simulink model "Scenario_17_v2"  (R2020b)
settings: Solver=ode1  StartTime=0.0  StopTime=10  FixedStep=Ts  MaxStep=Ts  MinStep=Ts/50  RelTol=1e-3
values from neighbouring files (symbols this model uses):
  c0 = c0_zeb    (= 6.57988e-09)    [Scenario_17_parameters_v2.m]    (also in Scenario_1_parameters_v2.m; Scenario_2_parameters_v2.m; Scenario_3_parameters_v2.m)
  c1 = c1_zeb    (= 9.15905e-09)    [Scenario_17_parameters_v2.m]    (also in Scenario_1_parameters_v2.m; Scenario_2_parameters_v2.m; Scenario_3_parameters_v2.m)
  fg = 50    [Scenario_17_parameters_v2.m]    (also in Scenario_1_parameters_v2.m; Scenario_2_parameters_v2.m; Scenario_3_parameters_v2.m)
  G11gen = 0.50    (= 0.5)    [Scenario_17_parameters_v2.m]
  G1gen = 0.4692    [Scenario_17_parameters_v2.m]    (also in Scenario_1_parameters_v2.m = 0.1; Scenario_2_parameters_v2.m = 0.298581; Scenario_3_parameters_v2.m = 0.65)
  G5gen = 0.75    [Scenario_17_parameters_v2.m]    (also in Scenario_1_parameters_v2.m = 0.8; Scenario_2_parameters_v2.m = 0.8; Scenario_3_parameters_v2.m = 0.705)
  G6gen = 0.90    (= 0.9)    [Scenario_17_parameters_v2.m]    (also in Scenario_1_parameters_v2.m; Scenario_2_parameters_v2.m = 0.81797; Scenario_3_parameters_v2.m = 0.45)
  G7gen = 0.20    (= 0.2)    [Scenario_17_parameters_v2.m]    (also in Scenario_1_parameters_v2.m = 0.5227; Scenario_2_parameters_v2.m = 0.5098; Scenario_3_parameters_v2.m = 0.4)
  G8gen = 0.58    [Scenario_17_parameters_v2.m]    (also in Scenario_3_parameters_v2.m = 0.65)
  G9gen = 0.8833    [Scenario_17_parameters_v2.m]    (also in Scenario_3_parameters_v2.m = 0.9)
  Iovc = 1.2    [Scenario_17_parameters_v2.m]    (also in Scenario_1_parameters_v2.m; Scenario_2_parameters_v2.m; Scenario_3_parameters_v2.m)
  l0 = l0_zeb    (= 0.00368)    [Scenario_17_parameters_v2.m]    (also in Scenario_1_parameters_v2.m; Scenario_2_parameters_v2.m; Scenario_3_parameters_v2.m)
  l1 = l1_zeb    (= 0.00128)    [Scenario_17_parameters_v2.m]    (also in Scenario_1_parameters_v2.m; Scenario_2_parameters_v2.m; Scenario_3_parameters_v2.m)
  L11dem = 0.02    [Scenario_17_parameters_v2.m]
  L12dem = 0.01    [Scenario_17_parameters_v2.m]    (also in Scenario_3_parameters_v2.m = 0.02)
  L1dem = 0.25    [Scenario_17_parameters_v2.m]    (also in Scenario_3_parameters_v2.m = 0.1)
  L3dem = 0.30    (= 0.3)    [Scenario_17_parameters_v2.m]    (also in Scenario_1_parameters_v2.m = 0.1; Scenario_2_parameters_v2.m = 0.1; Scenario_3_parameters_v2.m = 0.2)
  L5dem = 0.25    [Scenario_17_parameters_v2.m]    (also in Scenario_1_parameters_v2.m = 0.35; Scenario_2_parameters_v2.m = 0.35; Scenario_3_parameters_v2.m = 0.1)
  L9dem = 0.15    [Scenario_17_parameters_v2.m]    (also in Scenario_3_parameters_v2.m = 0.1)
  Pr = Sr*PF    (= 1600500000)    [Scenario_17_parameters_v2.m]    (also in Scenario_1_parameters_v2.m = 1472500000; Scenario_2_parameters_v2.m = 1805000000; Scenario_3_parameters_v2.m = 12740000000)
  Qr = sqrt(Sr^2 - Pr^2)    [Scenario_17_parameters_v2.m]    (also in Scenario_1_parameters_v2.m; Scenario_2_parameters_v2.m; Scenario_3_parameters_v2.m)
  r0 = r0_zeb    (= 0.39362)    [Scenario_17_parameters_v2.m]    (also in Scenario_1_parameters_v2.m; Scenario_2_parameters_v2.m; Scenario_3_parameters_v2.m)
  r1 = r1_zeb    (= 0.06862)    [Scenario_17_parameters_v2.m]    (also in Scenario_1_parameters_v2.m; Scenario_2_parameters_v2.m; Scenario_3_parameters_v2.m)
  Rtpu = Xtpu/40    (= 0.0025)    [Scenario_17_parameters_v2.m]    (also in Scenario_1_parameters_v2.m = 0.00375; Scenario_2_parameters_v2.m = 0.00375; Scenario_3_parameters_v2.m)
  S11non = 50e6    (= 50000000)    [Scenario_17_parameters_v2.m]
  S1non = 700e6    (= 700000000)    [Scenario_17_parameters_v2.m]    (also in Scenario_1_parameters_v2.m = 400000000; Scenario_2_parameters_v2.m = 400000000; Scenario_3_parameters_v2.m = 1000000000)
  S5non = 400e6    (= 400000000)    [Scenario_17_parameters_v2.m]    (also in Scenario_1_parameters_v2.m = 500000000; Scenario_2_parameters_v2.m = 500000000; Scenario_3_parameters_v2.m = 2000000000)
  S6non = 150e6    (= 150000000)    [Scenario_17_parameters_v2.m]    (also in Scenario_1_parameters_v2.m = 400000000; Scenario_2_parameters_v2.m = 400000000; Scenario_3_parameters_v2.m = 3000000000)
  S7non = 1500e6    (= 1500000000)    [Scenario_17_parameters_v2.m]    (also in Scenario_1_parameters_v2.m = 200000000; Scenario_2_parameters_v2.m = 200000000; Scenario_3_parameters_v2.m = 4000000000)
  S8non = 600e6    (= 600000000)    [Scenario_17_parameters_v2.m]    (also in Scenario_3_parameters_v2.m = 2000000000)
  S9non = 200e6    (= 200000000)    [Scenario_17_parameters_v2.m]    (also in Scenario_3_parameters_v2.m = 1500000000)
  tonvsc = 0    [Scenario_17_parameters_v2.m]    (also in Scenario_1_parameters_v2.m; Scenario_2_parameters_v2.m; Scenario_3_parameters_v2.m = 0.0001)
  Ts = 50e-6    (= 5e-05)    [Scenario_17_parameters_v2.m]    (also in Scenario_1_parameters_v2.m = 0.0002; Scenario_2_parameters_v2.m = 2e-05; Scenario_3_parameters_v2.m = 0.0001)
  Vhv = 220e3    (= 220000)    [Scenario_17_parameters_v2.m]    (also in Scenario_1_parameters_v2.m; Scenario_2_parameters_v2.m; Scenario_3_parameters_v2.m)
  Vmv = 22e3    (= 22000)    [Scenario_17_parameters_v2.m]    (also in Scenario_1_parameters_v2.m; Scenario_2_parameters_v2.m; Scenario_3_parameters_v2.m)
  w_pll = 2*pi*80    (= 502.654824574)    [Scenario_17_parameters_v2.m]    (also in Scenario_1_parameters_v2.m; Scenario_2_parameters_v2.m; Scenario_3_parameters_v2.m)
  wc1 = wsw1/10    (= 848.230016469)    [Scenario_17_parameters_v2.m]    (also in Scenario_1_parameters_v2.m; Scenario_2_parameters_v2.m; Scenario_3_parameters_v2.m)
  wdc1 = wc1/10    (= 84.8230016469)    [Scenario_17_parameters_v2.m]    (also in Scenario_1_parameters_v2.m; Scenario_2_parameters_v2.m; Scenario_3_parameters_v2.m)
  wpq1 = wc1/10    (= 84.8230016469)    [Scenario_17_parameters_v2.m]    (also in Scenario_1_parameters_v2.m; Scenario_2_parameters_v2.m; Scenario_3_parameters_v2.m)
  wsw1 = ksw1*2*pi*fg    (= 8482.30016469)    [Scenario_17_parameters_v2.m]    (also in Scenario_1_parameters_v2.m; Scenario_2_parameters_v2.m; Scenario_3_parameters_v2.m)
  Xtpu = 0.10    (= 0.1)    [Scenario_17_parameters_v2.m]    (also in Scenario_1_parameters_v2.m = 0.15; Scenario_2_parameters_v2.m = 0.15; Scenario_3_parameters_v2.m)
undefined symbols (not defined in the file or in its folder): D11, Delta, Newton, Raphson
libraries: powerlib x349, simulink_extras x215, powerlib_meascontrol x165, pid_lib x81, simulink x48, eeTransforms x42, spsFirstOrderFilterLib x28, eePwmGeneratorTwoLevel x7
(part 1 of 31)
settings Model: Creator=Usuario  LastModifiedBy=Usuario
settings SolverCC: InitialStep=Ts/50  MaxConsecutiveMinStep=100  ShapePreserveControl=EnableAll  ZeroCrossAlgorithm=Adaptive
settings DebuggingCC: UnconnectedInputMsg=none  UnconnectedOutputMsg=none  UnconnectedLineMsg=none

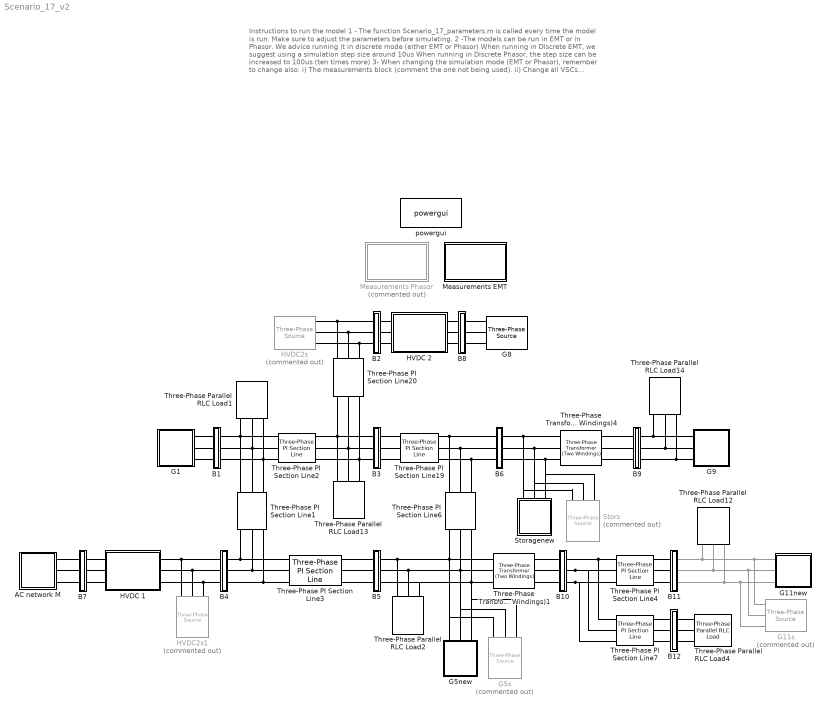
== system Scenario_17_v2 ==
  note: Instructions to run the model
      |
      | 1 - The function Scenario_17_parameters.m is called every time the model is run. Make sure to adjust the parameters before simulating.
      | 2 -The models can be run in EMT or in Phasor. We advice running it in discrete mode (either EMT or Phasor)
      | 	When running in Discrete EMT, we suggest using a simulation step size around 10us
      | 	When running in Discrete Phasor, the step size can be increased to 100us (ten times more)
      | 3- When changing the simulation mode (EMT or Phasor), remember to change also:
      | 	i) The measurements block (comment the one not being used).
      | 	ii) Change all VSCs models of blocks (G5,G11,Storage, HVDC 1 and HVDC 2).
      | 	    To change the model, go to the block VSC and choose one model of droplist under the parameter 'VSC model'
      | 	    We recommend the model AVG model for EMT and the I-ref model for Phasor.
      | 4- The synchronous generators were initialized using power flow to have a near-flat initialization.
      |      As the VSCs are not standard blocks in Simulink, they are not considered in the power flow.
      |     To consider them, connect the voltage source in their place and run the power flow. Then, substitute by the VSCs.
  AC network M : Subsystem
      mask Display: disp('SG')
  B1 : Subsystem
  B10 : Subsystem
  B11 : Subsystem
  B12 : Subsystem
  B2 : Subsystem
  B3 : Subsystem
  B4 : Subsystem
  B5 : Subsystem
  B6 : Subsystem
  B7 : Subsystem
  B8 : Subsystem
  B9 : Subsystem
  G1 : Subsystem
      mask Display:
      | disp('SG')
      | %x = [0:0.001:1];
      | %y = 0.2*sin(10*x) + 0.5;
      | %plot(x,y)
  G11new : Subsystem
  G11s : powerlib/Electrical Sources/Three-Phase Source  Commented=on  InternalConnection=Yg  VoltagePhases=off  Voltage=(22000)*1.15821  PhaseAngle=-42.2179  Voltage_phases=[25e3 25e3 25e3]/sqrt(3)  PhaseAngles_phases=[0 -120 +120]  Frequency=fg  NonIdealSource=on  SpecifyImpedance=off  Resistance=Rtpu*(Vmv^2/S11non)  Inductance=Xtpu*(Vmv^2/S11non) * 1/(2*pi*fg)  ShortCircuitLevel=Svsc1  BaseVoltage=Vmv  XRratio=Xtpu/Rtpu  BusType=PQ  Pref=S11non*G11gen  Qref=20e6  Prefabc=[10e3, 10e3, 10e3]  Qrefabc=[0, 0, 0]  Qmin=-inf  Qmax=inf
  G5new : Subsystem
  G5s : powerlib/Electrical Sources/Three-Phase Source  Commented=on  InternalConnection=Yg  VoltagePhases=off  Voltage=(220000)*1.07588  PhaseAngle=-28.957  Voltage_phases=[25e3 25e3 25e3]/sqrt(3)  PhaseAngles_phases=[0 -120 +120]  Frequency=fg  NonIdealSource=on  SpecifyImpedance=off  Resistance=Rtpu*(Vhv^2/S5non)  Inductance=Xtpu*(Vhv^2/S5non) * 1/(2*pi*fg)  ShortCircuitLevel=Svsc1  BaseVoltage=Vhv  XRratio=Xtpu/Rtpu  BusType=PQ  Pref=S5non*G5gen  Qref=150e6  Prefabc=[10e3, 10e3, 10e3]  Qrefabc=[0, 0, 0]  Qmin=-inf  Qmax=inf
  G8 : powerlib/Electrical Sources/Three-Phase Source  InternalConnection=Yg  VoltagePhases=off  Voltage=Vhv  PhaseAngle=0  Voltage_phases=[25e3 25e3 25e3]/sqrt(3)  PhaseAngles_phases=[0 -120 +120]  Frequency=fg  NonIdealSource=on  SpecifyImpedance=off  Resistance=Rtpu*(Vhv^2/S8non)  Inductance=Xtpu*(Vhv^2/S8non) * 1/(2*pi*fg)  ShortCircuitLevel=100e6  BaseVoltage=Vhv  XRratio=7  BusType=PV  Pref=S8non*G8gen  Qref=0  Prefabc=[10e3, 10e3, 10e3]  Qrefabc=[0, 0, 0]  Qmin=-inf  Qmax=inf
  G9 : Subsystem
      mask Display: disp('SG')
  HVDC 1 : Subsystem
  HVDC 2 : Subsystem
  HVDC2s : powerlib/Electrical Sources/Three-Phase Source  Commented=on  InternalConnection=Yg  VoltagePhases=off  Voltage=(220000)*0.984881  PhaseAngle=-24.9359  Voltage_phases=[25e3 25e3 25e3]/sqrt(3)  PhaseAngles_phases=[0 -120 +120]  Frequency=fg  NonIdealSource=on  SpecifyImpedance=off  Resistance=Rtpu*(Vhv^2/S8non)  Inductance=Xtpu*(Vhv^2/S8non) * 1/(2*pi*fg)  ShortCircuitLevel=Svsc1  BaseVoltage=Vhv  XRratio=Xtpu/Rtpu  BusType=PQ  Pref=S8non*G8gen  Qref=0  Prefabc=[10e3, 10e3, 10e3]  Qrefabc=[0, 0, 0]  Qmin=-inf  Qmax=inf
  HVDC2s1 : powerlib/Electrical Sources/Three-Phase Source  Commented=on  InternalConnection=Yg  VoltagePhases=off  Voltage=(220000)*1.05033  PhaseAngle=-28.8095  Voltage_phases=[25e3 25e3 25e3]/sqrt(3)  PhaseAngles_phases=[0 -120 +120]  Frequency=fg  NonIdealSource=on  SpecifyImpedance=off  Resistance=Rtpu*(Vhv^2/S7non)  Inductance=Xtpu*(Vhv^2/S7non) * 1/(2*pi*fg)  ShortCircuitLevel=Svsc1  BaseVoltage=Vhv  XRratio=Xtpu/Rtpu  BusType=PQ  Pref=S7non*G7gen  Qref=100e6  Prefabc=[10e3, 10e3, 10e3]  Qrefabc=[0, 0, 0]  Qmin=-inf  Qmax=inf
  Measurements EMT : Subsystem
  Measurements Phasor : Subsystem  Commented=on
  Storagenew : Subsystem
  Stors : powerlib/Electrical Sources/Three-Phase Source  Commented=on  InternalConnection=Yg  VoltagePhases=off  Voltage=(220000)*1.06618  PhaseAngle=-27.8909  Voltage_phases=[25e3 25e3 25e3]/sqrt(3)  PhaseAngles_phases=[0 -120 +120]  Frequency=fg  NonIdealSource=on  SpecifyImpedance=off  Resistance=Rtpu*(Vhv^2/S6non)  Inductance=Xtpu*(Vhv^2/S6non) * 1/(2*pi*fg)  ShortCircuitLevel=Svsc1  BaseVoltage=Vhv  XRratio=Xtpu/Rtpu  BusType=PQ  Pref=S6non*G6gen  Qref=80e6  Prefabc=[10e3, 10e3, 10e3]  Qrefabc=[0, 0, 0]  Qmin=-inf  Qmax=inf
  Three-Phase PI Section Line1 : powerlib/Elements/Three-Phase PI Section Line  LConnTagsString=a|b|c  RConnTagsString=A|B|C  Length=50  Frequency=fg  Resistances=[r1 r0]  Inductances="[l1  l0]"  Capacitances=[c1 c0]
  Three-Phase PI Section Line19 : powerlib/Elements/Three-Phase PI Section Line  LConnTagsString=a|b|c  RConnTagsString=A|B|C  Length=40  Frequency=fg  Resistances=[r1 r0]  Inductances="[l1  l0]"  Capacitances=[c1 c0]
  Three-Phase PI Section Line2 : powerlib/Elements/Three-Phase PI Section Line  LConnTagsString=a|b|c  RConnTagsString=A|B|C  Length=60  Frequency=fg  Resistances=[r1 r0]  Inductances="[l1  l0]"  Capacitances=[c1 c0]
  Three-Phase PI Section Line20 : powerlib/Elements/Three-Phase PI Section Line  LConnTagsString=a|b|c  RConnTagsString=A|B|C  Length=30  Frequency=fg  Resistances=[r1 r0]  Inductances="[l1  l0]"  Capacitances=[c1 c0]
  Three-Phase PI Section Line3 : powerlib/Elements/Three-Phase PI Section Line  LConnTagsString=a|b|c  RConnTagsString=A|B|C  Length=40  Frequency=fg  Resistances=[r1 r0]  Inductances="[l1  l0]"  Capacitances=[c1 c0]
  Three-Phase PI Section Line4 : powerlib/Elements/Three-Phase PI Section Line  LConnTagsString=a|b|c  RConnTagsString=A|B|C  Length=15  Frequency=fg  Resistances=[r1 r0]  Inductances="[l1  l0]"  Capacitances=[c1 c0]
  Three-Phase PI Section Line6 : powerlib/Elements/Three-Phase PI Section Line  LConnTagsString=a|b|c  RConnTagsString=A|B|C  Length=80  Frequency=fg  Resistances=[r1 r0]  Inductances="[l1  l0]"  Capacitances=[c1 c0]
  Three-Phase PI Section Line7 : powerlib/Elements/Three-Phase PI Section Line  LConnTagsString=a|b|c  RConnTagsString=A|B|C  Length=10  Frequency=fg  Resistances=[r1 r0]  Inductances="[l1  l0]"  Capacitances=[c1 c0]
  Three-Phase Parallel RLC Load1 : powerlib/Elements/Three-Phase Parallel RLC Load  LConnTagsString=A|B|C  Configuration=Y (grounded)  NominalVoltage=Vhv  Vabc=[1e3 1e3 1e3]  Vabcp=[1e3 1e3 1e3]  NominalFrequency=fg  UnbalancedPower=off  ActivePower=Pr*L1dem  InductivePower=Qr*L1dem  CapacitivePower=0  Pabc=[10e3 9e3 11e3]  QLabc=[100 90 110]  QCabc=[100 90 110]  Pabcp=[10e3 9e3 11e3]  QLabcp=[100 90 110]  QCabcp=[100 90 110]  Measurements=None  LoadType=constant Z
  Three-Phase Parallel RLC Load12 : powerlib/Elements/Three-Phase Parallel RLC Load  LConnTagsString=A|B|C  Configuration=Y (grounded)  NominalVoltage=Vmv  Vabc=[1e3 1e3 1e3]  Vabcp=[1e3 1e3 1e3]  NominalFrequency=fg  UnbalancedPower=off  ActivePower=Pr*L11dem  InductivePower=Qr*L11dem  CapacitivePower=0  Pabc=[10e3 9e3 11e3]  QLabc=[100 90 110]  QCabc=[100 90 110]  Pabcp=[10e3 9e3 11e3]  QLabcp=[100 90 110]  QCabcp=[100 90 110]  Measurements=None  LoadType=constant Z
  Three-Phase Parallel RLC Load13 : powerlib/Elements/Three-Phase Parallel RLC Load  LConnTagsString=A|B|C  Configuration=Y (grounded)  NominalVoltage=Vhv  Vabc=[1e3 1e3 1e3]  Vabcp=[1e3 1e3 1e3]  NominalFrequency=fg  UnbalancedPower=off  ActivePower=Pr*L3dem  InductivePower=Qr*L3dem  CapacitivePower=0  Pabc=[10e3 9e3 11e3]  QLabc=[100 90 110]  QCabc=[100 90 110]  Pabcp=[10e3 9e3 11e3]  QLabcp=[100 90 110]  QCabcp=[100 90 110]  Measurements=None  LoadType=constant Z
  Three-Phase Parallel RLC Load14 : powerlib/Elements/Three-Phase Parallel RLC Load  LConnTagsString=A|B|C  Configuration=Y (grounded)  NominalVoltage=Vmv  Vabc=[1e3 1e3 1e3]  Vabcp=[1e3 1e3 1e3]  NominalFrequency=fg  UnbalancedPower=off  ActivePower=Pr*L9dem  InductivePower=Qr*L9dem  CapacitivePower=0  Pabc=[10e3 9e3 11e3]  QLabc=[100 90 110]  QCabc=[100 90 110]  Pabcp=[10e3 9e3 11e3]  QLabcp=[100 90 110]  QCabcp=[100 90 110]  Measurements=None  LoadType=constant Z
  Three-Phase Parallel RLC Load2 : powerlib/Elements/Three-Phase Parallel RLC Load  LConnTagsString=A|B|C  Configuration=Y (grounded)  NominalVoltage=Vhv  Vabc=[1e3 1e3 1e3]  Vabcp=[1e3 1e3 1e3]  NominalFrequency=fg  UnbalancedPower=off  ActivePower=Pr*L5dem  InductivePower=Qr*L5dem  CapacitivePower=0  Pabc=[10e3 9e3 11e3]  QLabc=[100 90 110]  QCabc=[100 90 110]  Pabcp=[10e3 9e3 11e3]  QLabcp=[100 90 110]  QCabcp=[100 90 110]  Measurements=None  LoadType=constant Z
  Three-Phase Parallel RLC Load4 : powerlib/Elements/Three-Phase Parallel RLC Load  LConnTagsString=A|B|C  Configuration=Y (grounded)  NominalVoltage=Vmv  Vabc=[1e3 1e3 1e3]  Vabcp=[1e3 1e3 1e3]  NominalFrequency=fg  UnbalancedPower=off  ActivePower=Pr*L12dem  InductivePower=Qr*L12dem  CapacitivePower=0  Pabc=[10e3 9e3 11e3]  QLabc=[100 90 110]  QCabc=[100 90 110]  Pabcp=[10e3 9e3 11e3]  QLabcp=[100 90 110]  QCabcp=[100 90 110]  Measurements=None  LoadType=constant Z
  Three-Phase Transformer (Two Windings)1 : powerlib/Elements/Three-Phase Transformer (Two Windings)  Winding1Connection=Yg  Winding2Connection=Yg  CoreType=Three single-phase transformers  SetSaturation=off  Hysteresis=off  DataFile='hysteresis'  SetInitialFlux=off  Measurements=None  UNITS=pu  NominalPower=[2*S11non , fg ]  Winding1=[1.02*Vmv 0.001 0.04]  Winding2=[1.0*Vhv 0.001 0.04]  Rm=5000  Lm=5000  L0=0.5  Saturation=[ 0,0 ; 0.0024,1.2 ; 1.0,1.52 ]  InitialFluxes=[ 0.8 , -0.8 , 0.7 ]  BreakLoop=off  DiscreteSolver=Trapezoidal iterative  DataType=off  TransfoNumber=1
  Three-Phase Transformer (Two Windings)4 : powerlib/Elements/Three-Phase Transformer (Two Windings)  Winding1Connection=Yg  Winding2Connection=Yg  CoreType=Three single-phase transformers  SetSaturation=off  Hysteresis=off  DataFile='hysteresis'  SetInitialFlux=off  Measurements=None  UNITS=pu  NominalPower=[2*S9non , fg ]  Winding1=[1.0*Vmv 0.00125 0.05]  Winding2=[1.0*Vhv 0.00125 0.05]  Rm=5000  Lm=5000  L0=0.5  Saturation=[ 0,0 ; 0.0024,1.2 ; 1.0,1.52 ]  InitialFluxes=[ 0.8 , -0.8 , 0.7 ]  BreakLoop=off  DiscreteSolver=Trapezoidal iterative  DataType=off  TransfoNumber=1
  powergui : powerlib/powergui  Priority=1  SimulationMode=Discrete  SampleTime=Ts  frequency=fg  Iterations=50  frequencyindice=50  Pbase=100e6  ErrMax=0.0001  UnitsV=kV  UnitsW=MW  buscounter=0  FunctionMessages=off  echomessages=off  EnableUseOfTLC=off  CurrentSourceSwitches=off  DisableSnubberDevices=off  DisableRonSwitches=off  DisableVfSwitches=off  DisplayEquations=off  AutomaticDiscreteSolvers=off  SolverType=Tustin/Backward Euler (TBE)  Interpol=off  ExternalGateDelay=off  methode=off  Ts=100  x0status=blocks  SPID=on  SwTol=0  HookPort=off  NonlinearTolerance=1e-4  nMaxIteration=100  ContinueOnMaxIteration=off  RestoreLinks=warning  ResistiveCurrentMeasurement=off  Frange=[0:2:500]  Ylog=off  Xlog=on  ShowGrid=off  save=off  variable=ZData  structure=0  ZoomFFT=off  StartTime=0.0  cycles=1  DisplayStyle=1  fundamental=60  FreqAxis=off  MaxFrequency=1000  frequencyindicesteady=1  RmsSteady=2  display=off
  connections:
  B4/LConn1 -- HVDC 1/LConn1 -- HVDC2s1/RConn1
  B4/LConn2 -- HVDC2s1/RConn2 -- HVDC 1/LConn2
  B4/LConn3 -- HVDC2s1/RConn3 -- HVDC 1/LConn3
  G1/RConn1 -- B1/LConn1
  G1/RConn2 -- B1/LConn2
  G1/RConn3 -- B1/LConn3
  Three-Phase PI Section Line2/LConn1 -- Three-Phase Parallel RLC Load1/LConn1 -- Three-Phase PI Section Line1/RConn1 -- B1/RConn1
  Three-Phase PI Section Line2/LConn2 -- Three-Phase Parallel RLC Load1/LConn2 -- B1/RConn2 -- Three-Phase PI Section Line1/RConn2
  Three-Phase PI Section Line2/LConn3 -- B1/RConn3 -- Three-Phase Parallel RLC Load1/LConn3 -- Three-Phase PI Section Line1/RConn3
  Three-Phase PI Section Line3/LConn1 -- B4/RConn1 -- Three-Phase PI Section Line1/LConn1
  Three-Phase PI Section Line3/LConn2 -- B4/RConn2 -- Three-Phase PI Section Line1/LConn2
  Three-Phase PI Section Line3/LConn3 -- Three-Phase PI Section Line1/LConn3 -- B4/RConn3
  B5/LConn1 -- Three-Phase PI Section Line3/RConn1
  B5/LConn2 -- Three-Phase PI Section Line3/RConn2
  B5/LConn3 -- Three-Phase PI Section Line3/RConn3
  G5new/RConn1 -- G5s/RConn1 -- Three-Phase Transformer (Two Windings)1/RConn1 -- Three-Phase Parallel RLC Load2/LConn1 -- B5/RConn1 -- Three-Phase PI Section Line6/LConn1
  G5new/RConn2 -- G5s/RConn2 -- Three-Phase Parallel RLC Load2/LConn2 -- B5/RConn2 -- Three-Phase Transformer (Two Windings)1/RConn2 -- Three-Phase PI Section Line6/LConn2
  G5new/RConn3 -- G5s/RConn3 -- Three-Phase PI Section Line6/LConn3 -- Three-Phase Transformer (Two Windings)1/RConn3 -- Three-Phase Parallel RLC Load2/LConn3 -- B5/RConn3
  Three-Phase Transformer (Two Windings)1/LConn1 -- B10/LConn1
  Three-Phase Transformer (Two Windings)1/LConn2 -- B10/LConn2
  Three-Phase Transformer (Two Windings)1/LConn3 -- B10/LConn3
  Three-Phase PI Section Line7/LConn1 -- Three-Phase PI Section Line4/LConn1 -- B10/RConn1
  B10/RConn2 -- Three-Phase PI Section Line4/LConn2 -- Three-Phase PI Section Line7/LConn2
  B10/RConn3 -- Three-Phase PI Section Line4/LConn3 -- Three-Phase PI Section Line7/LConn3
  B12/LConn1 -- Three-Phase PI Section Line7/RConn1
  B12/LConn2 -- Three-Phase PI Section Line7/RConn2
  B12/LConn3 -- Three-Phase PI Section Line7/RConn3
  Three-Phase Parallel RLC Load4/LConn1 -- B12/RConn1
  Three-Phase Parallel RLC Load4/LConn2 -- B12/RConn2
  Three-Phase Parallel RLC Load4/LConn3 -- B12/RConn3
  Three-Phase PI Section Line4/RConn1 -- B11/LConn1
  Three-Phase PI Section Line4/RConn2 -- B11/LConn2
  Three-Phase PI Section Line4/RConn3 -- B11/LConn3
  G11s/RConn1 -- G11new/RConn1 -- Three-Phase Parallel RLC Load12/LConn1 -- B11/RConn1
  G11s/RConn3 -- G11new/RConn3 -- Three-Phase Parallel RLC Load12/LConn3 -- B11/RConn3
  G11s/RConn2 -- G11new/RConn2 -- Three-Phase Parallel RLC Load12/LConn2 -- B11/RConn2
  B3/LConn1 -- Three-Phase PI Section Line20/LConn1 -- Three-Phase Parallel RLC Load13/LConn1 -- Three-Phase PI Section Line2/RConn1
  B3/LConn2 -- Three-Phase PI Section Line20/LConn2 -- Three-Phase PI Section Line2/RConn2 -- Three-Phase Parallel RLC Load13/LConn2
  B3/LConn3 -- Three-Phase PI Section Line20/LConn3 -- Three-Phase Parallel RLC Load13/LConn3 -- Three-Phase PI Section Line2/RConn3
  Three-Phase PI Section Line19/LConn1 -- B3/RConn1
  Three-Phase PI Section Line19/LConn2 -- B3/RConn2
  Three-Phase PI Section Line19/LConn3 -- B3/RConn3
  Three-Phase PI Section Line19/RConn1 -- B6/LConn1 -- Three-Phase PI Section Line6/RConn1
  Three-Phase PI Section Line19/RConn2 -- Three-Phase PI Section Line6/RConn2 -- B6/LConn2
  Three-Phase PI Section Line19/RConn3 -- Three-Phase PI Section Line6/RConn3 -- B6/LConn3
  Three-Phase Transformer (Two Windings)4/RConn1 -- Stors/RConn1 -- Storagenew/RConn1 -- B6/RConn1
  Three-Phase Transformer (Two Windings)4/RConn2 -- Storagenew/RConn2 -- Stors/RConn2 -- B6/RConn2
  Three-Phase Transformer (Two Windings)4/RConn3 -- Storagenew/RConn3 -- Stors/RConn3 -- B6/RConn3
  B9/LConn1 -- Three-Phase Transformer (Two Windings)4/LConn1
  B9/LConn2 -- Three-Phase Transformer (Two Windings)4/LConn2
  B9/LConn3 -- Three-Phase Transformer (Two Windings)4/LConn3
  G9/RConn1 -- Three-Phase Parallel RLC Load14/LConn1 -- B9/RConn1
  G9/RConn2 -- Three-Phase Parallel RLC Load14/LConn2 -- B9/RConn2
  G9/RConn3 -- Three-Phase Parallel RLC Load14/LConn3 -- B9/RConn3
  HVDC 2/RConn3 -- B8/RConn3
  HVDC 2/RConn1 -- B8/RConn1
  G8/RConn1 -- B8/LConn1
  G8/RConn3 -- B8/LConn3
  G8/RConn2 -- B8/LConn2
  HVDC 2/RConn2 -- B8/RConn2
  HVDC 2/LConn1 -- B2/LConn1
  HVDC 2/LConn2 -- B2/LConn2
  HVDC 2/LConn3 -- B2/LConn3
  Three-Phase PI Section Line20/RConn1 -- HVDC2s/RConn1 -- B2/RConn1
  Three-Phase PI Section Line20/RConn2 -- HVDC2s/RConn2 -- B2/RConn2
  Three-Phase PI Section Line20/RConn3 -- HVDC2s/RConn3 -- B2/RConn3
  AC network M/RConn1 -- B7/LConn1
  AC network M/RConn2 -- B7/LConn2
  AC network M/RConn3 -- B7/LConn3
  HVDC 1/RConn1 -- B7/RConn1
  B7/RConn2 -- HVDC 1/RConn2
  HVDC 1/RConn3 -- B7/RConn3

== system Scenario_17_v2/AC network M ==
  note: Nomenclature (according to IEEE Std 421.1-2007):
      | Efd = Exciter output voltage (generator field voltage)
      | Ifd = Exciter output current (generator field current)
      | Vf = Excitation system stabilizer signal
      | Vfe = Signal proportional to exciter field current
      | Vl = Limiters and protective elements feedback
      | Vr = Regulator output
      | Vs = Power System Stabilizer (PSS) output
      | Vsi = Power System Stabilizer (PSS) inputs (shaft speed, frequency, generator electric power, and others
      | Vt = Generator terminal voltage
      | It = Generator terminal current
      | Vref = Voltage regulator reference signal
      | Vc = terminal voltage transducer output
  note: Synchronous Machine Model according to ENTSO-E
  Bus Selector : BusSelector  OutputSignals=dw,w,vq,vd,iq,id,Peo,Te
  Constant1 : Constant  Value=G7gen + 0.7 + 0.0082
  Exciter System : Subsystem
  Real-Imag to Complex : RealImagToComplex
  Real-Imag to Complex1 : RealImagToComplex
  Ref voltage (p.u) : Constant  Value=1.0
  SM : powerlib/Machines/Synchronous Machine pu Standard  PresetModel=No  MechanicalLoad=Mechanical power Pm  ShowDetailedParameters=on  RotorType=Salient-pole  Units=per unit standard parameters  MeasurementBus=on  NominalParameters=[S7non Vhv fg]  Reactances1=[ 1.81, 0.3, 0.23, 1.76, 0.65, 0.25, 0.15 ]  Reactances2=[2 0.35 0.25 1.8 0.3 0.15]  dAxisTimeConstants=Short-circuit  qAxisTimeConstants=Short-circuit  TimeConstants1="[ 4.4849  0.0681  0.1  ]"  TimeConstants2=[ 8.0, 0.03, 1.0, 0.07 ]  TimeConstants3="[  4.49  0.0681  0.0513  ]"  TimeConstants4=[ 8.0, 0.03, 0.3371, 0.0295 ]  TimeConstants5=[ 1.01, 0.053, 0.1 ]  TimeConstants6=[ 1.3201, 0.023, 1.0, 0.07 ]  TimeConstants7=[0.9 0.03 0.05]  TimeConstants8=[ 1.3201, 0.0231, 0.3371, 0.0295 ]  StatorResistance=0.01  Mechanical=[6 0 2]  PolePairs=20  InitialConditions=[0 -31.9163 0.9 0.9 0.9 1.66146e-14 -120 120 2.06132]  SetSaturation=off  Saturation=[0.6404,0.7127,0.8441,0.9214,0.9956,1.082,1.19,1.316,1.457;0.7,0.7698,0.8872,0.9466,0.9969,1.046,1.1,1.151,1.201]  LoadFlowParameters=[2 47500000 0 0 0]  TsPowergui=0  TsBlock=-1  IterativeModel=Trapezoidal non iterative  IterativeDiscreteModel=Trapezoidal non iterative  BusType=swing  Pref=475e6  Qref=0  Qmin=-inf  Qmax=inf  PLF=0  QLF=0
  Snubber : powerlib/Elements/Three-Phase Parallel RLC Load  LConnTagsString=A|B|C  Configuration=Y (grounded)  NominalVoltage=Vhv  Vabc=[1 1 1]*Vmv  Vabcp=[1e3 1e3 1e3]  NominalFrequency=fg  UnbalancedPower=off  ActivePower=0.7*S7non  InductivePower=0  CapacitivePower=0  Pabc=[10e3 10e3 10e3]  QLabc=[0 0 0]  QCabc=[0 0 0]  Pabcp=[10e3 9e3 11e3]  QLabcp=[100 90 110]  QCabcp=[100 90 110]  Measurements=None  LoadType=constant Z
  Speed Governor : Subsystem  mask{R=0.05, T1=0.5, T2=3, T3=10, Dt=0, Vmin=0, Vmax=10, P0=G7gen + 0.7 + 0.0082}
      mask prompts: R "Controller droop (R)"; T1 "Governor time constant (T1)(sec)"; T2 "Turbine derivative time constant (T2)(sec)"; T3 "Turbine delay time constant (T3)(sec)"; Dt "Frictional losses factor (Dt)"; Vmin "Minimum gate limit (Vmin)(p.u)"; Vmax "Maximum gate limit (Vmax)(p.u)"; P0 "Initial power (p.u)"
      mask Display:
      | disp('TGOV')
      | 
      | port_label('input',1,'Pref')
      | port_label('input',2,'dw')
      | 
      | port_label('output',1,'Pm')
  A : PMIOPort  Side=Right
  B : PMIOPort  Port=2  Side=Right
  C : PMIOPort  Port=3  Side=Right
  tag scope: Te7=global, wm7=global
  wires:
  Bus Selector/2 -> [wm7]  "<w>"
  Bus Selector/7 -> Exciter System/5(<Peo>)  "<Peo>"
  Real-Imag to Complex1/1 -> Exciter System/4(It)
  Real-Imag to Complex/1 -> Exciter System/3(Vt)
  Bus Selector/6 -> Real-Imag to Complex1/2  "<id>"
  Bus Selector/5 -> Real-Imag to Complex1/1  "<iq>"
  Bus Selector/3 -> Real-Imag to Complex/1  "<vq>"
  Bus Selector/4 -> Real-Imag to Complex/2  "<vd>"
  Bus Selector/1 -> Speed Governor/2(dw), Exciter System/1(<dw>)  "<dw>"
  SM/1 -> Bus Selector/1
  Exciter System/1(Efd) -> SM/2
  Ref voltage (p.u)/1 -> Exciter System/2(Vref)
  Speed Governor/1(Pm) -> SM/1
  Constant1/1 -> Speed Governor/1(RefL)
  Bus Selector/8 -> [Te7]  "<Te>"
  connections:
  Snubber/LConn2 -- B/RConn1 -- SM/RConn2
  Snubber/LConn3 -- C/RConn1 -- SM/RConn3
  Snubber/LConn1 -- A/RConn1 -- SM/RConn1

== system Scenario_17_v2/B1 ==
  Current Measurement : powerlib/Measurements/Current Measurement  PhasorSimulation=off  OutputType=Complex  PSBequivalent=0
  Current Measurement1 : powerlib/Measurements/Current Measurement  PhasorSimulation=off  OutputType=Complex  PSBequivalent=0
  Current Measurement2 : powerlib/Measurements/Current Measurement  PhasorSimulation=off  OutputType=Complex  PSBequivalent=0
  Gain : Gain
  Gain1 : Gain
  Ground : powerlib/Elements/Ground  LConnTagsString=a
  Ground1 : powerlib/Elements/Ground  LConnTagsString=a
  Ground2 : powerlib/Elements/Ground  LConnTagsString=a
  Load Flow Bus : powerlib/Measurements/Load Flow Bus  LConnTagsString=a  Phases=single  Connectors=on one side  ID=BUS1  Vbase=Vhv  Vref=1  Vangle=0  VLF=0.9929  VLFb=1  VLFc=1  angleLF=-32.51  angleLFb=0  angleLFc=0
  Mux : Mux  Inputs=3
  Mux1 : Mux  Inputs=3
  Voltage Measurement : powerlib/Measurements/Voltage Measurement  PhasorSimulation=off  OutputType=Complex  PSBequivalent=0
  Voltage Measurement1 : powerlib/Measurements/Voltage Measurement  PhasorSimulation=off  OutputType=Complex  PSBequivalent=0
  Voltage Measurement2 : powerlib/Measurements/Voltage Measurement  PhasorSimulation=off  OutputType=Complex  PSBequivalent=0
  A : PMIOPort  Side=Left
  B : PMIOPort  Port=2  Side=Left
  C : PMIOPort  Port=3  Side=Left
  a : PMIOPort  Port=4  Side=Right
  b : PMIOPort  Port=5  Side=Right
  c : PMIOPort  Port=6  Side=Right
  tag scope: I1=global, V1=global
  wires:
  Voltage Measurement2/1 -> Mux/3
  Voltage Measurement1/1 -> Mux/2
  Voltage Measurement/1 -> Mux/1
  Current Measurement/1 -> Mux1/1
  Current Measurement1/1 -> Mux1/2
  Current Measurement2/1 -> Mux1/3
  Mux/1 -> Gain/1
  Gain/1 -> [V1]
  Mux1/1 -> Gain1/1
  Gain1/1 -> [I1]
  connections:
  Current Measurement/RConn1 -- a/RConn1
  Current Measurement1/LConn1 -- Voltage Measurement1/LConn1 -- B/RConn1
  Current Measurement2/LConn1 -- Voltage Measurement2/LConn1 -- C/RConn1
  Current Measurement/LConn1 -- Voltage Measurement/LConn1 -- Load Flow Bus/LConn1 -- A/RConn1
  Current Measurement1/RConn1 -- b/RConn1
  Current Measurement2/RConn1 -- c/RConn1
  Ground/LConn1 -- Voltage Measurement/LConn2
  Ground1/LConn1 -- Voltage Measurement1/LConn2
  Ground2/LConn1 -- Voltage Measurement2/LConn2

== system Scenario_17_v2/B10 ==
  Current Measurement : powerlib/Measurements/Current Measurement  PhasorSimulation=off  OutputType=Complex  PSBequivalent=0
  Current Measurement1 : powerlib/Measurements/Current Measurement  PhasorSimulation=off  OutputType=Complex  PSBequivalent=0
  Current Measurement2 : powerlib/Measurements/Current Measurement  PhasorSimulation=off  OutputType=Complex  PSBequivalent=0
  Gain : Gain
  Gain1 : Gain
  Ground : powerlib/Elements/Ground  LConnTagsString=a
  Ground1 : powerlib/Elements/Ground  LConnTagsString=a
  Ground2 : powerlib/Elements/Ground  LConnTagsString=a
  Load Flow Bus : powerlib/Measurements/Load Flow Bus  LConnTagsString=a  Phases=single  Connectors=on one side  ID=BUS10  Vbase=Vmv  Vref=1  Vangle=0  VLF=1.056  VLFb=1  VLFc=1  angleLF=-34.13  angleLFb=0  angleLFc=0
  Mux : Mux  Inputs=3
  Mux1 : Mux  Inputs=3
  Voltage Measurement : powerlib/Measurements/Voltage Measurement  PhasorSimulation=off  OutputType=Complex  PSBequivalent=0
  Voltage Measurement1 : powerlib/Measurements/Voltage Measurement  PhasorSimulation=off  OutputType=Complex  PSBequivalent=0
  Voltage Measurement2 : powerlib/Measurements/Voltage Measurement  PhasorSimulation=off  OutputType=Complex  PSBequivalent=0
  A : PMIOPort  Side=Left
  B : PMIOPort  Port=2  Side=Left
  C : PMIOPort  Port=3  Side=Left
  a : PMIOPort  Port=4  Side=Right
  b : PMIOPort  Port=5  Side=Right
  c : PMIOPort  Port=6  Side=Right
  tag scope: I10=global, V10=global
  wires:
  Voltage Measurement2/1 -> Mux/3
  Voltage Measurement1/1 -> Mux/2
  Voltage Measurement/1 -> Mux/1
  Current Measurement/1 -> Mux1/1
  Current Measurement1/1 -> Mux1/2
  Current Measurement2/1 -> Mux1/3
  Mux/1 -> Gain/1
  Gain/1 -> [V10]
  Mux1/1 -> Gain1/1
  Gain1/1 -> [I10]
  connections:
  Current Measurement/RConn1 -- a/RConn1
  Current Measurement1/LConn1 -- Voltage Measurement1/LConn1 -- B/RConn1
  Current Measurement2/LConn1 -- Voltage Measurement2/LConn1 -- C/RConn1
  Current Measurement/LConn1 -- Voltage Measurement/LConn1 -- Load Flow Bus/LConn1 -- A/RConn1
  Current Measurement1/RConn1 -- b/RConn1
  Current Measurement2/RConn1 -- c/RConn1
  Ground/LConn1 -- Voltage Measurement/LConn2
  Ground1/LConn1 -- Voltage Measurement1/LConn2
  Ground2/LConn1 -- Voltage Measurement2/LConn2

== system Scenario_17_v2/B11 ==
  Current Measurement : powerlib/Measurements/Current Measurement  PhasorSimulation=off  OutputType=Complex  PSBequivalent=0
  Current Measurement1 : powerlib/Measurements/Current Measurement  PhasorSimulation=off  OutputType=Complex  PSBequivalent=0
  Current Measurement2 : powerlib/Measurements/Current Measurement  PhasorSimulation=off  OutputType=Complex  PSBequivalent=0
  Gain : Gain
  Gain1 : Gain
  Ground : powerlib/Elements/Ground  LConnTagsString=a
  Ground1 : powerlib/Elements/Ground  LConnTagsString=a
  Ground2 : powerlib/Elements/Ground  LConnTagsString=a
  Load Flow Bus : powerlib/Measurements/Load Flow Bus  LConnTagsString=a  Phases=single  Connectors=on one side  ID=BUS11  Vbase=Vmv  Vref=1  Vangle=0  VLF=1.121  VLFb=1  VLFc=1  angleLF=-44.38  angleLFb=0  angleLFc=0
  Mux : Mux  Inputs=3
  Mux1 : Mux  Inputs=3
  Voltage Measurement : powerlib/Measurements/Voltage Measurement  PhasorSimulation=off  OutputType=Complex  PSBequivalent=0
  Voltage Measurement1 : powerlib/Measurements/Voltage Measurement  PhasorSimulation=off  OutputType=Complex  PSBequivalent=0
  Voltage Measurement2 : powerlib/Measurements/Voltage Measurement  PhasorSimulation=off  OutputType=Complex  PSBequivalent=0
  A : PMIOPort  Side=Left
  B : PMIOPort  Port=2  Side=Left
  C : PMIOPort  Port=3  Side=Left
  a : PMIOPort  Port=4  Side=Right
  b : PMIOPort  Port=5  Side=Right
  c : PMIOPort  Port=6  Side=Right
  tag scope: I11=global, V11=global
  wires:
  Voltage Measurement2/1 -> Mux/3
  Voltage Measurement1/1 -> Mux/2
  Voltage Measurement/1 -> Mux/1
  Current Measurement/1 -> Mux1/1
  Current Measurement1/1 -> Mux1/2
  Current Measurement2/1 -> Mux1/3
  Mux/1 -> Gain/1
  Gain/1 -> [V11]
  Mux1/1 -> Gain1/1
  Gain1/1 -> [I11]
  connections:
  Current Measurement/RConn1 -- a/RConn1
  Current Measurement1/LConn1 -- Voltage Measurement1/LConn1 -- B/RConn1
  Current Measurement2/LConn1 -- Voltage Measurement2/LConn1 -- C/RConn1
  Current Measurement/LConn1 -- Voltage Measurement/LConn1 -- Load Flow Bus/LConn1 -- A/RConn1
  Current Measurement1/RConn1 -- b/RConn1
  Current Measurement2/RConn1 -- c/RConn1
  Ground/LConn1 -- Voltage Measurement/LConn2
  Ground1/LConn1 -- Voltage Measurement1/LConn2
  Ground2/LConn1 -- Voltage Measurement2/LConn2

== system Scenario_17_v2/B12 ==
  Current Measurement : powerlib/Measurements/Current Measurement  PhasorSimulation=off  OutputType=Complex  PSBequivalent=0
  Current Measurement1 : powerlib/Measurements/Current Measurement  PhasorSimulation=off  OutputType=Complex  PSBequivalent=0
  Current Measurement2 : powerlib/Measurements/Current Measurement  PhasorSimulation=off  OutputType=Complex  PSBequivalent=0
  Gain : Gain
  Gain1 : Gain
  Ground : powerlib/Elements/Ground  LConnTagsString=a
  Ground1 : powerlib/Elements/Ground  LConnTagsString=a
  Ground2 : powerlib/Elements/Ground  LConnTagsString=a
  Load Flow Bus : powerlib/Measurements/Load Flow Bus  LConnTagsString=a  Phases=single  Connectors=on one side  ID=BUS12  Vbase=Vmv  Vref=1  Vangle=0  VLF=0.9925  VLFb=1  VLFc=1  angleLF=-41.01  angleLFb=0  angleLFc=0
  Mux : Mux  Inputs=3
  Mux1 : Mux  Inputs=3
  Voltage Measurement : powerlib/Measurements/Voltage Measurement  PhasorSimulation=off  OutputType=Complex  PSBequivalent=0
  Voltage Measurement1 : powerlib/Measurements/Voltage Measurement  PhasorSimulation=off  OutputType=Complex  PSBequivalent=0
  Voltage Measurement2 : powerlib/Measurements/Voltage Measurement  PhasorSimulation=off  OutputType=Complex  PSBequivalent=0
  A : PMIOPort  Side=Left
  B : PMIOPort  Port=2  Side=Left
  C : PMIOPort  Port=3  Side=Left
  a : PMIOPort  Port=4  Side=Right
  b : PMIOPort  Port=5  Side=Right
  c : PMIOPort  Port=6  Side=Right
  tag scope: I12=global, V12=global
  wires:
  Voltage Measurement2/1 -> Mux/3
  Voltage Measurement1/1 -> Mux/2
  Voltage Measurement/1 -> Mux/1
  Current Measurement/1 -> Mux1/1
  Current Measurement1/1 -> Mux1/2
  Current Measurement2/1 -> Mux1/3
  Mux/1 -> Gain/1
  Gain/1 -> [V12]
  Mux1/1 -> Gain1/1
  Gain1/1 -> [I12]
  connections:
  Current Measurement/RConn1 -- a/RConn1
  Current Measurement1/LConn1 -- Voltage Measurement1/LConn1 -- B/RConn1
  Current Measurement2/LConn1 -- Voltage Measurement2/LConn1 -- C/RConn1
  Current Measurement/LConn1 -- Voltage Measurement/LConn1 -- Load Flow Bus/LConn1 -- A/RConn1
  Current Measurement1/RConn1 -- b/RConn1
  Current Measurement2/RConn1 -- c/RConn1
  Ground/LConn1 -- Voltage Measurement/LConn2
  Ground1/LConn1 -- Voltage Measurement1/LConn2
  Ground2/LConn1 -- Voltage Measurement2/LConn2

== system Scenario_17_v2/B2 ==
  Current Measurement : powerlib/Measurements/Current Measurement  PhasorSimulation=off  OutputType=Complex  PSBequivalent=0
  Current Measurement1 : powerlib/Measurements/Current Measurement  PhasorSimulation=off  OutputType=Complex  PSBequivalent=0
  Current Measurement2 : powerlib/Measurements/Current Measurement  PhasorSimulation=off  OutputType=Complex  PSBequivalent=0
  Gain : Gain
  Gain1 : Gain
  Ground : powerlib/Elements/Ground  LConnTagsString=a
  Ground1 : powerlib/Elements/Ground  LConnTagsString=a
  Ground2 : powerlib/Elements/Ground  LConnTagsString=a
  Load Flow Bus : powerlib/Measurements/Load Flow Bus  LConnTagsString=a  Phases=single  Connectors=on one side  ID=BUS2  Vbase=Vhv  Vref=1  Vangle=0  VLF=0.9816  VLFb=1  VLFc=1  angleLF=-28.38  angleLFb=0  angleLFc=0
  Mux : Mux  Inputs=3
  Mux1 : Mux  Inputs=3
  Voltage Measurement : powerlib/Measurements/Voltage Measurement  PhasorSimulation=off  OutputType=Complex  PSBequivalent=0
  Voltage Measurement1 : powerlib/Measurements/Voltage Measurement  PhasorSimulation=off  OutputType=Complex  PSBequivalent=0
  Voltage Measurement2 : powerlib/Measurements/Voltage Measurement  PhasorSimulation=off  OutputType=Complex  PSBequivalent=0
  A : PMIOPort  Side=Left
  B : PMIOPort  Port=2  Side=Left
  C : PMIOPort  Port=3  Side=Left
  a : PMIOPort  Port=4  Side=Right
  b : PMIOPort  Port=5  Side=Right
  c : PMIOPort  Port=6  Side=Right
  tag scope: I2=global, V2=global
  wires:
  Voltage Measurement2/1 -> Mux/3
  Voltage Measurement1/1 -> Mux/2
  Voltage Measurement/1 -> Mux/1
  Current Measurement/1 -> Mux1/1
  Current Measurement1/1 -> Mux1/2
  Current Measurement2/1 -> Mux1/3
  Mux/1 -> Gain/1
  Gain/1 -> [V2]
  Mux1/1 -> Gain1/1
  Gain1/1 -> [I2]
  connections:
  Current Measurement/RConn1 -- a/RConn1
  Current Measurement1/LConn1 -- Voltage Measurement1/LConn1 -- B/RConn1
  Current Measurement2/LConn1 -- Voltage Measurement2/LConn1 -- C/RConn1
  Current Measurement/LConn1 -- Voltage Measurement/LConn1 -- Load Flow Bus/LConn1 -- A/RConn1
  Current Measurement1/RConn1 -- b/RConn1
  Current Measurement2/RConn1 -- c/RConn1
  Ground/LConn1 -- Voltage Measurement/LConn2
  Ground1/LConn1 -- Voltage Measurement1/LConn2
  Ground2/LConn1 -- Voltage Measurement2/LConn2

== system Scenario_17_v2/B3 ==
  Current Measurement : powerlib/Measurements/Current Measurement  PhasorSimulation=off  OutputType=Complex  PSBequivalent=0
  Current Measurement1 : powerlib/Measurements/Current Measurement  PhasorSimulation=off  OutputType=Complex  PSBequivalent=0
  Current Measurement2 : powerlib/Measurements/Current Measurement  PhasorSimulation=off  OutputType=Complex  PSBequivalent=0
  Gain : Gain
  Gain1 : Gain
  Ground : powerlib/Elements/Ground  LConnTagsString=a
  Ground1 : powerlib/Elements/Ground  LConnTagsString=a
  Ground2 : powerlib/Elements/Ground  LConnTagsString=a
  Load Flow Bus : powerlib/Measurements/Load Flow Bus  LConnTagsString=a  Phases=single  Connectors=on one side  ID=BUS3  Vbase=Vhv  Vref=1  Vangle=0  VLF=0.9701  VLFb=1  VLFc=1  angleLF=-33.6  angleLFb=0  angleLFc=0
  Mux : Mux  Inputs=3
  Mux1 : Mux  Inputs=3
  Voltage Measurement : powerlib/Measurements/Voltage Measurement  PhasorSimulation=off  OutputType=Complex  PSBequivalent=0
  Voltage Measurement1 : powerlib/Measurements/Voltage Measurement  PhasorSimulation=off  OutputType=Complex  PSBequivalent=0
  Voltage Measurement2 : powerlib/Measurements/Voltage Measurement  PhasorSimulation=off  OutputType=Complex  PSBequivalent=0
  A : PMIOPort  Side=Left
  B : PMIOPort  Port=2  Side=Left
  C : PMIOPort  Port=3  Side=Left
  a : PMIOPort  Port=4  Side=Right
  b : PMIOPort  Port=5  Side=Right
  c : PMIOPort  Port=6  Side=Right
  tag scope: I3=global, V3=global
  wires:
  Voltage Measurement2/1 -> Mux/3
  Voltage Measurement1/1 -> Mux/2
  Voltage Measurement/1 -> Mux/1
  Current Measurement/1 -> Mux1/1
  Current Measurement1/1 -> Mux1/2
  Current Measurement2/1 -> Mux1/3
  Mux/1 -> Gain/1
  Gain/1 -> [V3]
  Mux1/1 -> Gain1/1
  Gain1/1 -> [I3]
  connections:
  Current Measurement/RConn1 -- a/RConn1
  Current Measurement1/LConn1 -- Voltage Measurement1/LConn1 -- B/RConn1
  Current Measurement2/LConn1 -- Voltage Measurement2/LConn1 -- C/RConn1
  Current Measurement/LConn1 -- Voltage Measurement/LConn1 -- Load Flow Bus/LConn1 -- A/RConn1
  Current Measurement1/RConn1 -- b/RConn1
  Current Measurement2/RConn1 -- c/RConn1
  Ground/LConn1 -- Voltage Measurement/LConn2
  Ground1/LConn1 -- Voltage Measurement1/LConn2
  Ground2/LConn1 -- Voltage Measurement2/LConn2

== system Scenario_17_v2/B4 ==
  Current Measurement : powerlib/Measurements/Current Measurement  PhasorSimulation=off  OutputType=Complex  PSBequivalent=0
  Current Measurement1 : powerlib/Measurements/Current Measurement  PhasorSimulation=off  OutputType=Complex  PSBequivalent=0
  Current Measurement2 : powerlib/Measurements/Current Measurement  PhasorSimulation=off  OutputType=Complex  PSBequivalent=0
  Gain : Gain
  Gain1 : Gain
  Ground : powerlib/Elements/Ground  LConnTagsString=a
  Ground1 : powerlib/Elements/Ground  LConnTagsString=a
  Ground2 : powerlib/Elements/Ground  LConnTagsString=a
  Load Flow Bus : powerlib/Measurements/Load Flow Bus  LConnTagsString=a  Phases=single  Connectors=on one side  ID=BUS4  Vbase=Vhv  Vref=1  Vangle=0  VLF=1.043  VLFb=1  VLFc=1  angleLF=-29.85  angleLFb=0  angleLFc=0
  Mux : Mux  Inputs=3
  Mux1 : Mux  Inputs=3
  Voltage Measurement : powerlib/Measurements/Voltage Measurement  PhasorSimulation=off  OutputType=Complex  PSBequivalent=0
  Voltage Measurement1 : powerlib/Measurements/Voltage Measurement  PhasorSimulation=off  OutputType=Complex  PSBequivalent=0
  Voltage Measurement2 : powerlib/Measurements/Voltage Measurement  PhasorSimulation=off  OutputType=Complex  PSBequivalent=0
  A : PMIOPort  Side=Left
  B : PMIOPort  Port=2  Side=Left
  C : PMIOPort  Port=3  Side=Left
  a : PMIOPort  Port=4  Side=Right
  b : PMIOPort  Port=5  Side=Right
  c : PMIOPort  Port=6  Side=Right
  tag scope: I4=global, V4=global
  wires:
  Voltage Measurement2/1 -> Mux/3
  Voltage Measurement1/1 -> Mux/2
  Voltage Measurement/1 -> Mux/1
  Current Measurement/1 -> Mux1/1
  Current Measurement1/1 -> Mux1/2
  Current Measurement2/1 -> Mux1/3
  Mux/1 -> Gain/1
  Gain/1 -> [V4]
  Mux1/1 -> Gain1/1
  Gain1/1 -> [I4]
  connections:
  Current Measurement/RConn1 -- a/RConn1
  Current Measurement1/LConn1 -- Voltage Measurement1/LConn1 -- B/RConn1
  Current Measurement2/LConn1 -- Voltage Measurement2/LConn1 -- C/RConn1
  Current Measurement/LConn1 -- Voltage Measurement/LConn1 -- Load Flow Bus/LConn1 -- A/RConn1
  Current Measurement1/RConn1 -- b/RConn1
  Current Measurement2/RConn1 -- c/RConn1
  Ground/LConn1 -- Voltage Measurement/LConn2
  Ground1/LConn1 -- Voltage Measurement1/LConn2
  Ground2/LConn1 -- Voltage Measurement2/LConn2

== system Scenario_17_v2/B5 ==
  Current Measurement : powerlib/Measurements/Current Measurement  PhasorSimulation=off  OutputType=Complex  PSBequivalent=0
  Current Measurement1 : powerlib/Measurements/Current Measurement  PhasorSimulation=off  OutputType=Complex  PSBequivalent=0
  Current Measurement2 : powerlib/Measurements/Current Measurement  PhasorSimulation=off  OutputType=Complex  PSBequivalent=0
  Gain : Gain
  Gain1 : Gain
  Ground : powerlib/Elements/Ground  LConnTagsString=a
  Ground1 : powerlib/Elements/Ground  LConnTagsString=a
  Ground2 : powerlib/Elements/Ground  LConnTagsString=a
  Load Flow Bus : powerlib/Measurements/Load Flow Bus  LConnTagsString=a  Phases=single  Connectors=on one side  ID=BUS5  Vbase=Vhv  Vref=1  Vangle=0  VLF=1.035  VLFb=1  VLFc=1  angleLF=-32.77  angleLFb=0  angleLFc=0
  Mux : Mux  Inputs=3
  Mux1 : Mux  Inputs=3
  Voltage Measurement : powerlib/Measurements/Voltage Measurement  PhasorSimulation=off  OutputType=Complex  PSBequivalent=0
  Voltage Measurement1 : powerlib/Measurements/Voltage Measurement  PhasorSimulation=off  OutputType=Complex  PSBequivalent=0
  Voltage Measurement2 : powerlib/Measurements/Voltage Measurement  PhasorSimulation=off  OutputType=Complex  PSBequivalent=0
  A : PMIOPort  Side=Left
  B : PMIOPort  Port=2  Side=Left
  C : PMIOPort  Port=3  Side=Left
  a : PMIOPort  Port=4  Side=Right
  b : PMIOPort  Port=5  Side=Right
  c : PMIOPort  Port=6  Side=Right
  tag scope: I5=global, V5=global
  wires:
  Voltage Measurement2/1 -> Mux/3
  Voltage Measurement1/1 -> Mux/2
  Voltage Measurement/1 -> Mux/1
  Current Measurement/1 -> Mux1/1
  Current Measurement1/1 -> Mux1/2
  Current Measurement2/1 -> Mux1/3
  Mux/1 -> Gain/1
  Gain/1 -> [V5]
  Mux1/1 -> Gain1/1
  Gain1/1 -> [I5]
  connections:
  Current Measurement/RConn1 -- a/RConn1
  Current Measurement1/LConn1 -- Voltage Measurement1/LConn1 -- B/RConn1
  Current Measurement2/LConn1 -- Voltage Measurement2/LConn1 -- C/RConn1
  Current Measurement/LConn1 -- Voltage Measurement/LConn1 -- Load Flow Bus/LConn1 -- A/RConn1
  Current Measurement1/RConn1 -- b/RConn1
  Current Measurement2/RConn1 -- c/RConn1
  Ground/LConn1 -- Voltage Measurement/LConn2
  Ground1/LConn1 -- Voltage Measurement1/LConn2
  Ground2/LConn1 -- Voltage Measurement2/LConn2

== system Scenario_17_v2/B6 ==
  Current Measurement : powerlib/Measurements/Current Measurement  PhasorSimulation=off  OutputType=Complex  PSBequivalent=0
  Current Measurement1 : powerlib/Measurements/Current Measurement  PhasorSimulation=off  OutputType=Complex  PSBequivalent=0
  Current Measurement2 : powerlib/Measurements/Current Measurement  PhasorSimulation=off  OutputType=Complex  PSBequivalent=0
  Gain : Gain
  Gain1 : Gain
  Ground : powerlib/Elements/Ground  LConnTagsString=a
  Ground1 : powerlib/Elements/Ground  LConnTagsString=a
  Ground2 : powerlib/Elements/Ground  LConnTagsString=a
  Load Flow Bus : powerlib/Measurements/Load Flow Bus  LConnTagsString=a  Phases=single  Connectors=on one side  ID=BUS6  Vbase=Vhv  Vref=1  Vangle=0  VLF=1.007  VLFb=1  VLFc=1  angleLF=-32.63  angleLFb=0  angleLFc=0
  Mux : Mux  Inputs=3
  Mux1 : Mux  Inputs=3
  Voltage Measurement : powerlib/Measurements/Voltage Measurement  PhasorSimulation=off  OutputType=Complex  PSBequivalent=0
  Voltage Measurement1 : powerlib/Measurements/Voltage Measurement  PhasorSimulation=off  OutputType=Complex  PSBequivalent=0
  Voltage Measurement2 : powerlib/Measurements/Voltage Measurement  PhasorSimulation=off  OutputType=Complex  PSBequivalent=0
  A : PMIOPort  Side=Left
  B : PMIOPort  Port=2  Side=Left
  C : PMIOPort  Port=3  Side=Left
  a : PMIOPort  Port=4  Side=Right
  b : PMIOPort  Port=5  Side=Right
  c : PMIOPort  Port=6  Side=Right
  tag scope: I6=global, V6=global
  wires:
  Voltage Measurement2/1 -> Mux/3
  Voltage Measurement1/1 -> Mux/2
  Voltage Measurement/1 -> Mux/1
  Current Measurement/1 -> Mux1/1
  Current Measurement1/1 -> Mux1/2
  Current Measurement2/1 -> Mux1/3
  Mux/1 -> Gain/1
  Gain/1 -> [V6]
  Mux1/1 -> Gain1/1
  Gain1/1 -> [I6]
  connections:
  Current Measurement/RConn1 -- a/RConn1
  Current Measurement1/LConn1 -- Voltage Measurement1/LConn1 -- B/RConn1
  Current Measurement2/LConn1 -- Voltage Measurement2/LConn1 -- C/RConn1
  Current Measurement/LConn1 -- Voltage Measurement/LConn1 -- Load Flow Bus/LConn1 -- A/RConn1
  Current Measurement1/RConn1 -- b/RConn1
  Current Measurement2/RConn1 -- c/RConn1
  Ground/LConn1 -- Voltage Measurement/LConn2
  Ground1/LConn1 -- Voltage Measurement1/LConn2
  Ground2/LConn1 -- Voltage Measurement2/LConn2
